simulink model "opamp_analysis"  (R2024a)
settings: Solver=VariableStepAuto  StartTime=0.0  StopTime=simlength  RelTol=1e-3
undefined symbols (not defined in the file): a_uin, f_uin
libraries: fl_lib x12, nesl_utility x4, ee_lib x2, opamp_lib x1
settings Model: Creator=dbagn  LastModifiedBy=dbagn

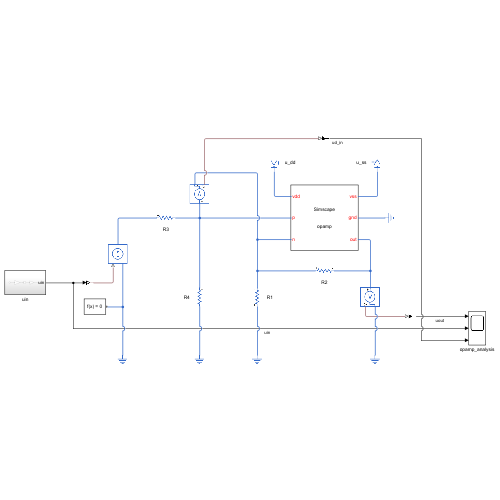
[thumbnail: Simulink's stored preview of the top-level diagram]
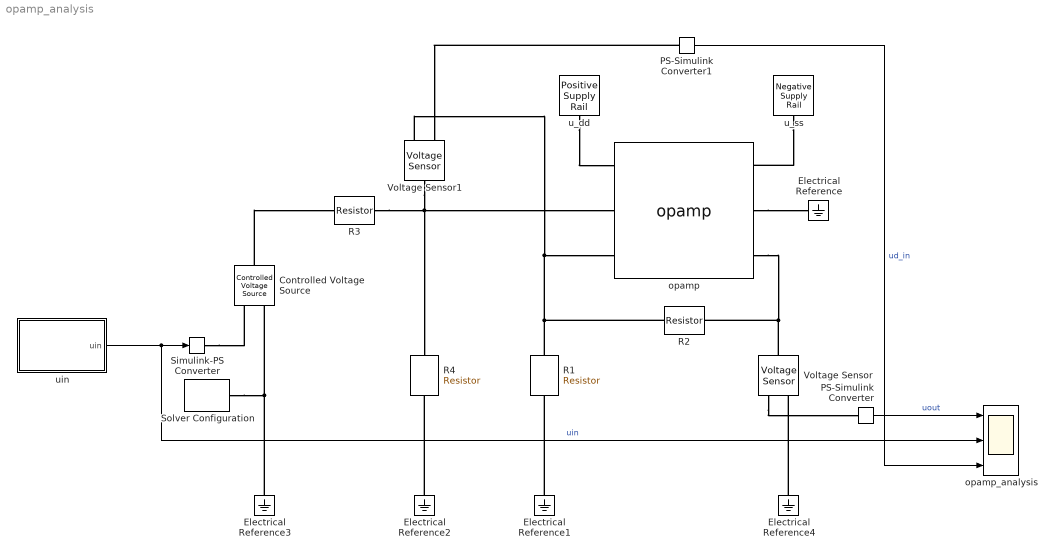
== system opamp_analysis ==
  Controlled Voltage Source : fl_lib/Electrical/Electrical Sources/Controlled Voltage Source
  Electrical Reference{,1..4} (5 alike) : fl_lib/Electrical/Electrical Elements/Electrical Reference
  PS-Simulink Converter : nesl_utility/PS-Simulink Converter  PhysicalDomain=network_engine_domain  SubClassName=ps_output  LeftPortType=input  RightPortType=output  PseudoPeriodic=off  Frequencies=[]  VectorFormat=1-D array  Unit=V  AffineConversion=off
  PS-Simulink Converter1 : nesl_utility/PS-Simulink Converter  PhysicalDomain=network_engine_domain  SubClassName=ps_output  LeftPortType=input  RightPortType=output  PseudoPeriodic=off  Frequencies=[]  VectorFormat=1-D array  Unit=V  AffineConversion=off
  R{1..4} (4 alike) : fl_lib/Electrical/Electrical Elements/Resistor  R=1e3 Ohm  i_specify=off  i_priority=None  i=0 A  i_nominal_specify=off  i_nominal_value=1  i_nominal_unit=A  v_specify=off  v_priority=None  v=0 V  v_nominal_specify=off  v_nominal_value=1  v_nominal_unit=V
  Simulink-PS Converter : nesl_utility/Simulink-PS Converter  PhysicalDomain=network_engine_domain  SubClassName=ps_input  LeftPortType=input  RightPortType=output  PseudoPeriodic=off  Frequencies=[]  NoiseDistribution=none  NoiseParameters=[]  Unit=V  AffineConversion=off  FilteringAndDerivatives=provide  SimscapeFilterOrder=1  InputFilterTimeConstant=0.001  UdotUserProvided=0
  Solver Configuration : nesl_utility/Solver Configuration  PhysicalDomain=network_engine_domain  SubClassName=solver  LeftPortType=input  RightPortType=generic  Tones=[]  Harmonics=[]  SimulateNoise=off  Profile=off  UseLocalSampling=off  EnableSwitchedLinearOptims=on  FrequencyDomain=off  UseCCode=off  RelTol=0.001  AbsTol=0.001  MinStep=1e-09  ToWorkspace=off  RevertToSquareIcSolve=off  NumHomotopyIterations=100  PhasorMode=off  PhasorModeNumHarmonics=1  ConsistencySolver=NEWTON_XTOL_AFTER_FTOL  IndexReductionMethod=DerivativeReplacement  DoDC=on  ResidualTolerance=1e-09  ConsistencyTolSource=GLOBAL  ConsistencyAbsTol=0.001  ConsistencyRelTol=0.001  ConsistencyTolFactor=0.001  UseLocalSolver=on  LocalSolverChoice=NE_BACKWARD_EULER_ADVANCER  ResolveIndetEquations=on  FunctionEvalNumThread=1  LocalSolverSampleTime=tc  DoFixedCost=on  MaxNonlinIter=3  MaxModeIter=2  ComputeImpulses=off  ImpulseIterations=2  LinearAlgebra=auto  LinearAlgebraNumThread=0  EquationFormulation=NE_TIME_EF  DelaysMemoryBudget=1024  AutomaticFiltering=on  FilteringTimeConstant=0.001  PartitionStorageMethod=AS_NEEDED  PartitionMemoryBudget=1024  PartitionMethod=ROBUST  MultibodyUseLocalSolver=off  MultibodyLocalSolverChoice=ODE1  MultibodyLocalSolverSampleTime=0.001
  Voltage Sensor : fl_lib/Electrical/Electrical Sensors/Voltage Sensor
  Voltage Sensor1 : fl_lib/Electrical/Electrical Sensors/Voltage Sensor
  opamp : opamp_lib/opamp  Rin=1e4 Ohm  Rout=1 Ohm  A=1e5  Acm=1  vgamma=0.7 V  Rb=1 Ohm  id_specify=off  id_priority=None  id=0 A  id_nominal_specify=off  id_nominal_value=1  id_nominal_unit=A  vd_specify=off  vd_priority=None  vd=0 V  vd_nominal_specify=off  vd_nominal_value=1  vd_nominal_unit=V  i_out_specify=off  i_out_priority=None  i_out=0 A  i_out_nominal_specify=off  i_out_nominal_value=1  i_out_nominal_unit=A  vm_specify=off  vm_priority=None  vm=0 V  vm_nominal_specify=off  vm_nominal_value=1  vm_nominal_unit=V  v_out_specify=off  v_out_priority=None  v_out=0 V  v_out_nominal_specify=off  v_out_nominal_value=1  v_out_nominal_unit=V  vdd_s_specify=off  vdd_s_priority=None  vdd_s=0 V  vdd_s_nominal_specify=off  vdd_s_nominal_value=1  vdd_s_nominal_unit=V  vss_s_specify=off  vss_s_priority=None  vss_s=0 V  vss_s_nominal_specify=off  vss_s_nominal_value=1  vss_s_nominal_unit=V
      settings: InternalSimscapePortConfiguration="{\"Bottom\":[],\"Left\":[{\"id\":\"vdd\",\"label\":\"vdd\",\"type\":\"foundation.electrical.electrical\"},{\"id\":\"p\",\"label\":\"p\",\"type\":\"foundation.electrical.electrical\"},{\"id\":\"n\",\"label\":\"n\",\"type\":\"foundation.electrical.electrical\"}],\"Right\":[{\"id\":\"vss\",\"label\":\"vss\",\"type\":\"foundation.electrical.electrical\"},{\"id\":\"gnd\",\"label\":\"gnd\",\"type\":\"foundation.electrical.electrical\"},{\"id\":\"out\",\"label\":\"out\",\"type\":\"foundation.electrical.electrical\"}],\"Top\":[]}"
  opamp_analysis : Scope  NumInputPorts=3
  u_dd : ee_lib/Sources/Positive Supply Rail  v0=u_dd V
      settings: InternalSimscapePortConfiguration="{\"Bottom\":[],\"Left\":[],\"Right\":[{\"id\":\"p\",\"label\":\"\",\"type\":\"foundation.electrical.electrical\"}],\"Top\":[]}"
  u_ss : ee_lib/Sources/Negative Supply Rail  v0=u_ss V
      settings: InternalSimscapePortConfiguration="{\"Bottom\":[],\"Left\":[{\"id\":\"n\",\"label\":\"\",\"type\":\"foundation.electrical.electrical\"}],\"Right\":[],\"Top\":[]}"
  uin : Subsystem
  wires:
  PS-Simulink Converter/1 -> opamp_analysis/1  "uout"
  PS-Simulink Converter1/1 -> opamp_analysis/3  "ud_in"
  uin/1(uin) -> opamp_analysis/2, Simulink-PS Converter/1  "uin"
  connections:
  u_dd/RConn1 -- opamp/LConn1
  u_ss/LConn1 -- opamp/RConn1
  opamp/RConn2 -- Electrical Reference/LConn1
  opamp/RConn3 -- Voltage Sensor/LConn1 -- R2/RConn1
  Electrical Reference1/LConn1 -- R1/LConn1
  R3/RConn1 -- opamp/LConn2 -- R4/LConn1 -- Voltage Sensor1/LConn1
  Electrical Reference2/LConn1 -- R4/RConn1
  R1/RConn1 -- R2/LConn1 -- opamp/LConn3 -- Voltage Sensor1/RConn2
  Controlled Voltage Source/LConn1 -- R3/LConn1
  Simulink-PS Converter/RConn1 -- Controlled Voltage Source/RConn1
  Electrical Reference3/LConn1 -- Solver Configuration/RConn1 -- Controlled Voltage Source/RConn2
  Voltage Sensor/RConn1 -- PS-Simulink Converter/LConn1
  Electrical Reference4/LConn1 -- Voltage Sensor/RConn2
  PS-Simulink Converter1/LConn1 -- Voltage Sensor1/RConn1

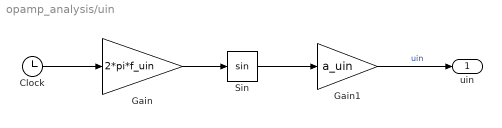
== system opamp_analysis/uin ==
  Clock : Clock
  Gain : Gain  Gain=2*pi*f_uin
  Gain1 : Gain  Gain=a_uin
  Sin : Trigonometry
  uin : Outport
  wires:
  Sin/1 -> Gain1/1
  Clock/1 -> Gain/1
  Gain/1 -> Sin/1
  Gain1/1 -> uin/1  "uin"
